simulink model "state_space_seesaw_matlabsimulink_29_04_2024"  (R2023b)
settings: Solver=VariableStepAuto  StartTime=0.0  StopTime=30  FixedStep=3  RelTol=1e-3
values from neighbouring files (symbols this model uses):
  A = [0,mf*g*h/Jconst,0,-mf*g/Jconst; 1,0,0,0; 0,-g,0,0; 0,0,1,0]    [state_space_seesaw_matlabsimulink_29_04_2024_inizalise.m]
  B = [1/Jconst;0;0;0]    [state_space_seesaw_matlabsimulink_29_04_2024_inizalise.m]
  g = 9.81    [state_space_seesaw_matlabsimulink_29_04_2024_inizalise.m]
  h = 0.1    [state_space_seesaw_matlabsimulink_29_04_2024_inizalise.m]
  Jconst = mf*h^2+Jb    (= 0.501)    [state_space_seesaw_matlabsimulink_29_04_2024_inizalise.m]
  kT = qT*(alpha(5)*eye(4)+alpha(4)*A+alpha(3)*A^2+alpha(2)*A^3+A^4)    [state_space_seesaw_matlabsimulink_29_04_2024_inizalise.m]
  mf = 0.1    [state_space_seesaw_matlabsimulink_29_04_2024_inizalise.m]
  P = 1/(C*inv(B*kT-A)*B)    [state_space_seesaw_matlabsimulink_29_04_2024_inizalise.m]
settings Model: Creator=dmplab  LastModifiedBy=Krish
settings DebuggingCC: UnconnectedInputMsg=warning  UnconnectedOutputMsg=warning  UnconnectedLineMsg=warning
settings ModelReferenceCC: EnableRefExpFcnMdlSchedulingChecks=on
settings RTWCC: DLArmComputeVersion=19.05

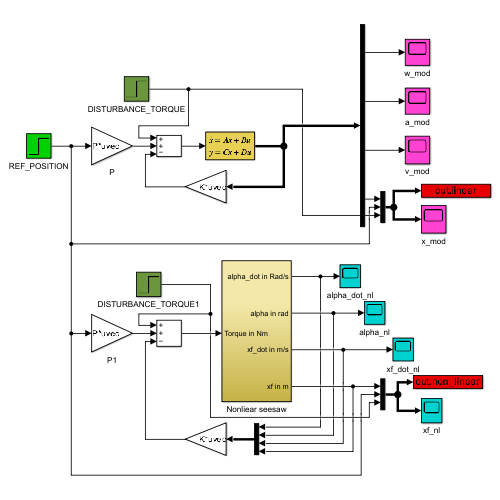
[thumbnail: Simulink's stored preview of the top-level diagram]
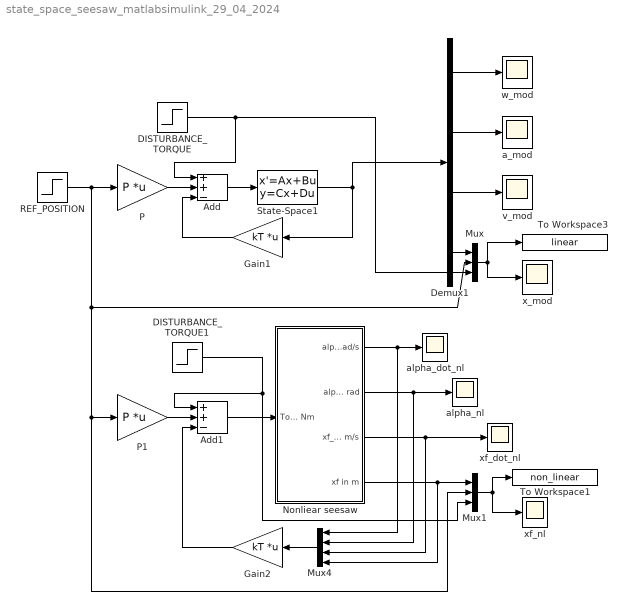
== system state_space_seesaw_matlabsimulink_29_04_2024 ==
  Add : Sum  Inputs=++-
  Add1 : Sum  Inputs=++-
  DISTURBANCE_TORQUE : Step  Time=15  After=0.1  SampleTime=0
  DISTURBANCE_TORQUE1 : Step  Time=15  After=0.1  SampleTime=0
  Demux1 : Demux
  Gain1 : Gain  Gain=kT  Multiplication=Matrix(K*u) (u vector)
  Gain2 : Gain  Gain=kT  Multiplication=Matrix(K*u) (u vector)
  Mux : Mux  Inputs=3
  Mux1 : Mux  Inputs=3
  Mux4 : Mux
  Nonliear seesaw : Subsystem
  P : Gain  Gain=P  Multiplication=Matrix(K*u) (u vector)
  P1 : Gain  Gain=P  Multiplication=Matrix(K*u) (u vector)
  REF_POSITION : Step  SampleTime=0
  State-Space1 : StateSpace  A=A  B=B  C=eye(4)  D=[0;0;0;0]  InitialCondition=0
  To Workspace1 : ToWorkspace  VariableName=non_linear  SaveFormat=Timeseries  SampleTime=-1
  To Workspace3 : ToWorkspace  VariableName=linear  SaveFormat=Timeseries  SampleTime=-1
  a_mod : Scope
  alpha_dot_nl : Scope
  alpha_nl : Scope
  v_mod : Scope
  w_mod : Scope
  x_mod : Scope
  xf_dot_nl : Scope
  xf_nl : Scope
  wires:
  P/1 -> Add/2
  Add/1 -> State-Space1/1
  Gain1/1 -> Add/3
  State-Space1/1 -> Gain1/1, Demux1/1
  Demux1/1 -> w_mod/1
  Demux1/4 -> Mux/1
  Mux/1 -> To Workspace3/1, x_mod/1
  Demux1/2 -> a_mod/1
  Demux1/3 -> v_mod/1
  DISTURBANCE_TORQUE/1 -> Add/1, Mux/3
  Nonliear seesaw/1(alpha_dot in Rad/s) -> Mux4/1, alpha_dot_nl/1
  Nonliear seesaw/3(xf_dot in m/s) -> Mux4/3, xf_dot_nl/1
  Add1/1 -> Nonliear seesaw/1(Torque in Nm)
  Nonliear seesaw/4(xf in m) -> Mux4/4, Mux1/1
  Nonliear seesaw/2(alpha in rad) -> Mux4/2, alpha_nl/1
  P1/1 -> Add1/2
  Gain2/1 -> Add1/3
  DISTURBANCE_TORQUE1/1 -> Mux1/3, Add1/1
  REF_POSITION/1 -> Mux1/2, P1/1, Mux/2, P/1
  Mux4/1 -> Gain2/1
  Mux1/1 -> To Workspace1/1, xf_nl/1

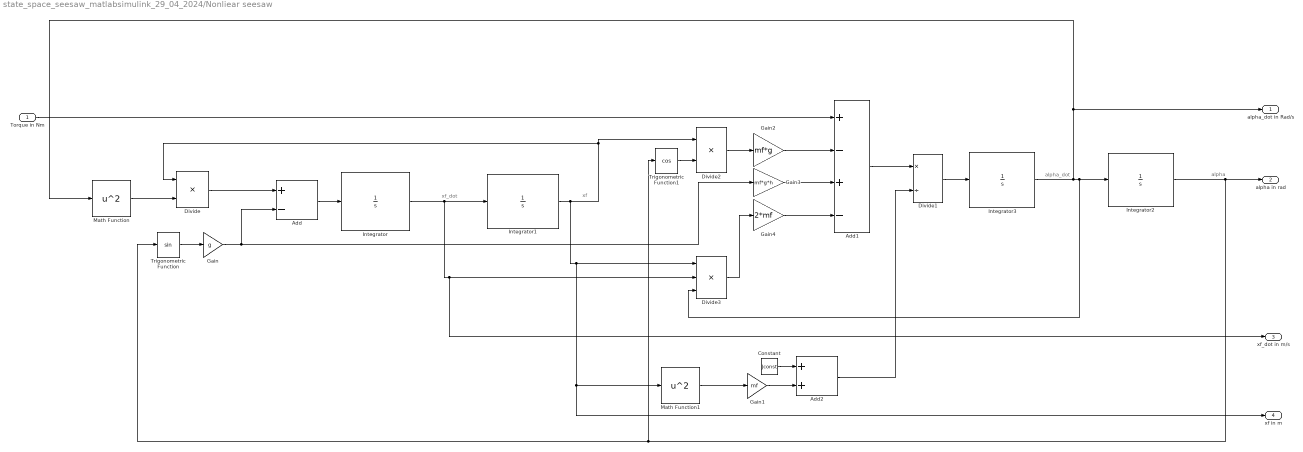
== system state_space_seesaw_matlabsimulink_29_04_2024/Nonliear seesaw ==
  note: alpha_dot
  note: xf_dot
  note: xf
  note: alpha
  Torque in Nm : Inport
  Add : Sum  Inputs=+-
  Add1 : Sum  Inputs=+-+-
  Add2 : Sum
  Constant : Constant  Value=Jconst
  Divide : Product  Inputs=**
  Divide1 : Product  Inputs=*/
  Divide2 : Product  Inputs=**
  Divide3 : Product  Inputs=***
  Gain : Gain  Gain=g
  Gain1 : Gain  Gain=mf
  Gain2 : Gain  Gain=mf*g
  Gain3 : Gain  Gain=mf*g*h
  Gain4 : Gain  Gain=2*mf
  Integrator{,1..3} (4 alike) : Integrator
  Math Function : Math  Operator=square
  Math Function1 : Math  Operator=square
  Trigonometric Function : Trigonometry
  Trigonometric Function1 : Trigonometry  Operator=cos
  alpha_dot in Rad/s : Outport
  alpha in rad : Outport  Port=2
  xf_dot in m/s : Outport  Port=3
  xf in m : Outport  Port=4
  wires:
  Gain/1 -> Gain3/1, Add/2
  Integrator2/1 -> Trigonometric Function1/1, Trigonometric Function/1, alpha in rad/1
  Integrator/1 -> xf_dot in m/s/1, Divide3/2, Integrator1/1
  Integrator3/1 -> Integrator2/1, Divide3/3, alpha_dot in Rad/s/1, Math Function/1
  Divide/1 -> Add/1
  Integrator1/1 -> xf in m/1, Math Function1/1, Divide3/1, Divide/1, Divide2/1
  Constant/1 -> Add2/1
  Divide3/1 -> Gain4/1
  Gain2/1 -> Add1/2
  Math Function/1 -> Divide/2
  Add/1 -> Integrator/1
  Gain4/1 -> Add1/4
  Gain1/1 -> Add2/2
  Trigonometric Function/1 -> Gain/1
  Math Function1/1 -> Gain1/1
  Add1/1 -> Divide1/1
  Gain3/1 -> Add1/3
  Divide1/1 -> Integrator3/1
  Add2/1 -> Divide1/2
  Divide2/1 -> Gain2/1
  Trigonometric Function1/1 -> Divide2/2
  Torque in Nm/1 -> Add1/1
